simulink subsystem "Controller"  (R2023b)
settings: Solver=VariableStepAuto  StartTime=0.0  StopTime=10.0  RelTol=1e-3
undefined symbols (not defined in the file): tActiveDischargeDelay, tCloseContDelay, tSim
libraries: simulink x1
settings Model: DataDictionary=ElectricPowertrain_data.sldd  EnableAccessToBaseWorkspace=off  Creator=Elio  LastModifiedBy=Elio

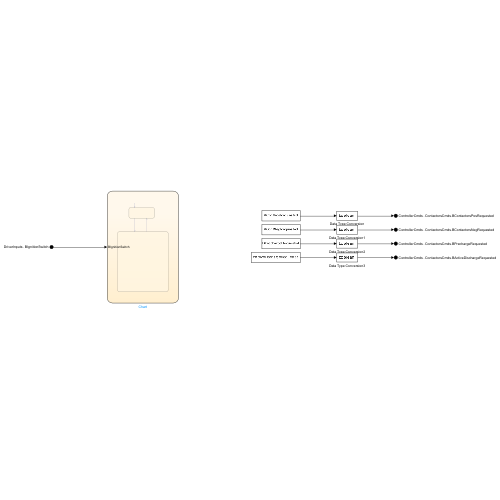
[thumbnail: Simulink's stored preview of the top-level diagram]
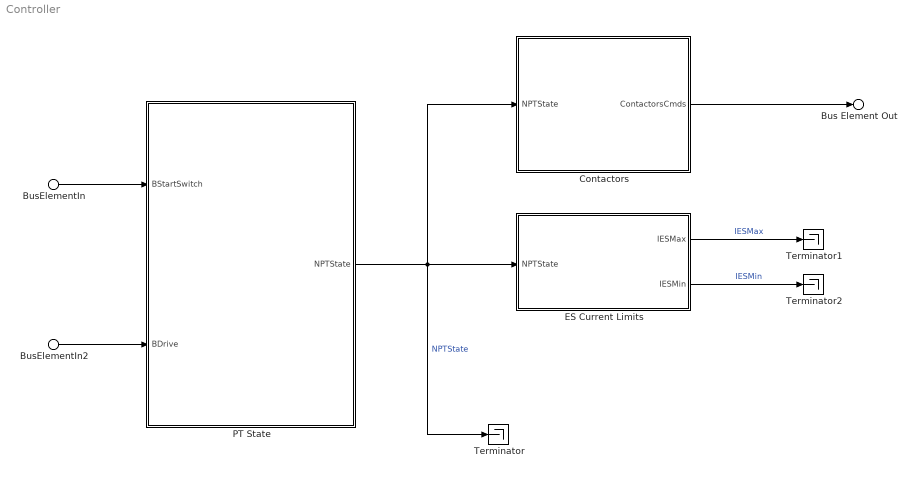
== system Controller ==
  BusElementIn : Inport  PortName=DriverCmds  Element=BStartSwitch
  BusElementIn2 : Inport  PortName=DriverCmds  Element=BDrive
  Contactors : Subsystem
  ES Current Limits : Subsystem
  PT State : Stateflow chart  TreatAsAtomicUnit=on
  Terminator : Terminator
  Terminator1 : Terminator
  Terminator2 : Terminator
  Bus Element Out : Outport  PortName=ControllerCmds  Element=ContactorsCmds
  wires:
  BusElementIn/1 -> PT State/1(BStartSwitch)
  PT State/1(NPTState) -> Contactors/1(NPTState), ES Current Limits/1(NPTState), Terminator/1  "NPTState"
  BusElementIn2/1 -> PT State/2(BDrive)
  Contactors/1(ContactorsCmds) -> Bus Element Out/1
  ES Current Limits/1(IESMax) -> Terminator1/1  "IESMax"
  ES Current Limits/2(IESMin) -> Terminator2/1  "IESMin"

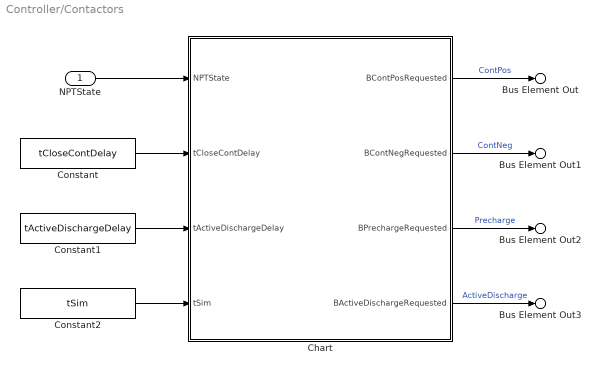
== system Controller/Contactors ==
  NPTState : Inport
  Chart : Stateflow chart  TreatAsAtomicUnit=on
      settings: PortSchema="{\"entries\":[{\"content\":{\"sides\":[{\"content\":{\"connectorIds\":[\"In1\",\"In2\",\"In3\",\"In4\"]},\"type\":\"ConnectorPlacement.EquallySpacedRectSide\",\"uuid\":\"5a0065c0-5db5-4462-bbdd-2fd5e45287aa\"},{\"content\":{\"connectorIds\":[\"Out2\",\"Out3\",\"Out1\",\"Out4\"],\"side\":\"RIGHT\"},\"type\":\"ConnectorPlacement.EquallySpacedRectSide\",\"uuid\":\"ede6eff5-c813-4ab8-91a1-3986418acd87\"},{\"content\":{\"side\":\"TOP\"},\"type\":\"ConnectorPlacement.EquallySpacedRectSide\",\"uuid\":\"7d6725e0-16fb-455f-af2a-820d6785b0ed\"}]},\"type\":\"ConnectorPlacement.EquallySpacedConnector\",\"uuid\":\"9151490c-92d8-4c01-9b8a-0e09fae469db\"}],\"packageUris\":[\"http://schema.mathworks.com/mf0/Connector/R2020b\"],\"version\":\"1.0\"}"
  Constant : Constant  Value=tCloseContDelay  SampleTime=tSim
  Constant1 : Constant  Value=tActiveDischargeDelay  SampleTime=tSim
  Constant2 : Constant  Value=tSim  SampleTime=tSim
  Bus Element Out : Outport  PortName=ContactorsCmds  Element=BContPosRequested
  Bus Element Out1 : Outport  PortName=ContactorsCmds  Element=BContNegRequested
  Bus Element Out2 : Outport  PortName=ContactorsCmds  Element=BPrechargeRequested
  Bus Element Out3 : Outport  PortName=ContactorsCmds  Element=BActiveDischargeRequested
  wires:
  Constant2/1 -> Chart/4(tSim)
  Constant1/1 -> Chart/3(tActiveDischargeDelay)
  Constant/1 -> Chart/2(tCloseContDelay)
  Chart/4(BActiveDischargeRequested) -> Bus Element Out3/1  "ActiveDischarge"
  Chart/3(BContNegRequested) -> Bus Element Out1/1  "ContNeg"
  Chart/2(BContPosRequested) -> Bus Element Out/1  "ContPos"
  Chart/1(BPrechargeRequested) -> Bus Element Out2/1  "Precharge"
  NPTState/1 -> Chart/1(NPTState)

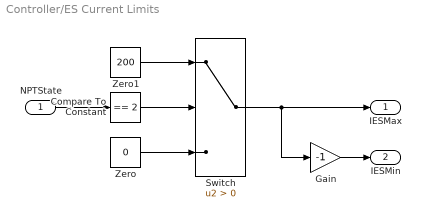
== system Controller/ES Current Limits ==
  NPTState : Inport
  Compare To Constant : simulink/Logic and Bit Operations/Compare To Constant  relop===  const=2  OutDataTypeStr=boolean
  Gain : Gain  Gain=-1
  Switch : Switch  Criteria=u2 > Threshold  SaturateOnIntegerOverflow=off  InputSameDT=off
  Zero : Constant  Value=0  OutDataTypeStr=Inherit: Inherit via back propagation  SampleTime=tSim
  Zero1 : Constant  Value=200  OutDataTypeStr=Inherit: Inherit via back propagation  SampleTime=tSim
  IESMax : Outport
  IESMin : Outport  Port=2
  wires:
  Gain/1 -> IESMin/1
  Switch/1 -> Gain/1, IESMax/1
  Zero1/1 -> Switch/1
  Zero/1 -> Switch/3
  Compare To Constant/1 -> Switch/2
  NPTState/1 -> Compare To Constant/1

== stateflow chart Controller/PT State ==
  state OFF
    NPTState = eNPTState.Off;
  state OPEN_CONTACTORS
    NPTState = eNPTState.OpenContactors;
  state ON
    state CLOSE_CONTACTORS
      NPTState = eNPTState.CloseContactors;
    state TORQUE_CONTROL
      NPTState = eNPTState.TorqueControl;
    (default) -> CLOSE_CONTACTORS
    CLOSE_CONTACTORS -> TORQUE_CONTROL : [BDrive]
    TORQUE_CONTROL -> CLOSE_CONTACTORS : [!BDrive]
  (default) -> OFF
  OPEN_CONTACTORS -> OFF
  (junction 34) -> OPEN_CONTACTORS
  OFF -> ON : [BStartSwitch]
  ON -> (junction 34) : [!BStartSwitch]
  data: BStartSwitch input; NPTState output double; BDrive input

== stateflow chart Controller/Contactors/Chart ==
  state STANDBY
    BContPosRequested = 0;
    BContNegRequested = 0;
    BPrechargeRequested = 0;
    BActiveDischargeRequested = 0;
    tDelay = 0;
  state CLOSE_SEQUENCE
    state CLOSE_PRECHARGE
      BPrechargeRequested = 1;
    state CLOSE_NEG
      BContNegRequested = 1;
    state CLOSE_POS
      BContPosRequested = 1;
    state OPEN_PRECHARGE
      BPrechargeRequested = 0;
    (default) -> CLOSE_PRECHARGE
    CLOSE_PRECHARGE -> (junction 53) : {tDelay += tSim;}
    (junction 53) -> CLOSE_NEG : [tDelay >= tCloseContDelay]
        | {tDelay = 0;}
    CLOSE_NEG -> (junction 57) : {tDelay += tSim;}
    (junction 57) -> CLOSE_POS : [tDelay >= tCloseContDelay]
        | {tDelay = 0;}
    CLOSE_POS -> (junction 60) : {tDelay += tSim;}
    (junction 60) -> OPEN_PRECHARGE : [tDelay >= tCloseContDelay]
        | {tDelay = 0;}
  state OPEN_SEQUENCE
    state OPEN_CONTACTORS
      BContPosRequested = 0;
      BContNegRequested = 0;
      BPrechargeRequested = 0;
      BActiveDischargeRequested = 1;
    (default) -> OPEN_CONTACTORS
    OPEN_CONTACTORS -> (junction 37) : {tDelay += tSim;}
    (junction 37) -> 46 : [tDelay >= tActiveDischargeDelay]
  (default) -> STANDBY
  (junction 28) -> STANDBY
  47 -> (junction 28)
  STANDBY -> CLOSE_SEQUENCE : [NPTState == 1]
  CLOSE_SEQUENCE -> OPEN_SEQUENCE : [NPTState == 3]
      | {tDelay = 0;}
  data: NPTState input; BPrechargeRequested output boolean; BContPosRequested output boolean; BContNegRequested output boolean; BActiveDischargeRequested output boolean; tCloseContDelay input; tActiveDischargeDelay input; tDelay local double; tSim input
